simulink library "lidar_script_other_ver"  (R2021a)
settings: Solver=VariableStepAuto  StartTime=0.0  StopTime=10.0  RelTol=1e-3
undefined symbols (not defined in the file or in its folder): sim3d
settings Model: ModifiedByFormat=The MathWorks, Inc.  Creator=The MathWorks, Inc.  LastModifiedBy=The MathWorks, Inc.
settings SolverCC: AlgebraicLoopSolver=TrustRegion
settings DebuggingCC: SFMachineParentedDataDiag=warning

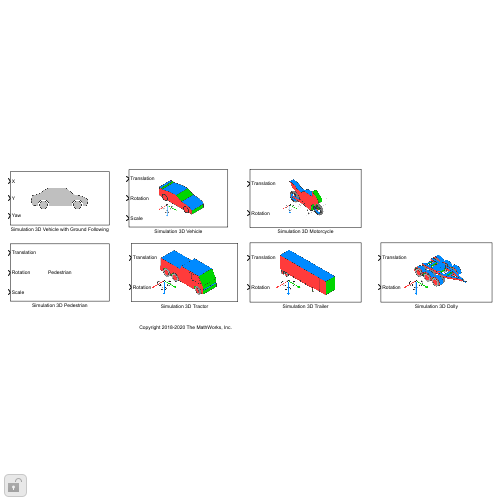
[thumbnail: Simulink's stored preview of the top-level diagram]
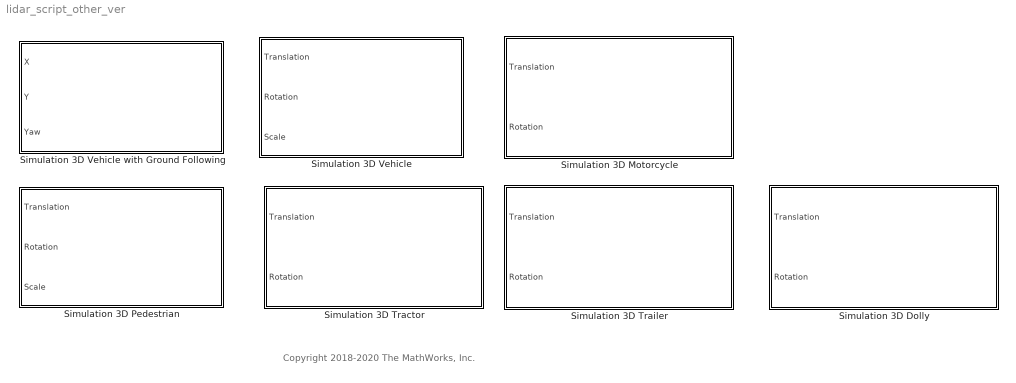
== system lidar_script_other_ver ==
  note: Copyright 2018-2020 The MathWorks, Inc.
  Simulation 3D Dolly : Subsystem  Priority=-1  LoadFcn=sim3d.SimPool.loadCallback(gcb)  mask(Simulation 3D Dolly){Mesh=One-axle dolly, Mesh_Internal=One-axle dolly, ActorName=, Translation=zeros( 5, 3 ), Rotation=zeros( 5, 3 ), Scale=ones( 5, 3 ), SampleTime=-1, ActorType=SimulinkVehicle, ID=[], aMode=aMode, ActorTag=}
      mask prompts: Mesh "shared_sim3dblks:sim3dblkDolly:blkPrm_Mesh"; Mesh_Internal "shared_sim3dblks:sim3dblkDolly:blkPrm_Mesh"; ActorName "shared_sim3dblks:sim3dblkDolly:blkPrm_ActorName"; Translation "shared_sim3dblks:sim3dblkDolly:blkPrm_Translation"; Rotation "shared_sim3dblks:sim3dblkDolly:blkPrm_Rotation"; SampleTime "shared_sim3dblks:sim3dblkDolly:blkPrm_SampleTime"
      mask help: shared_sim3dblks:sim3dblkDolly:blkDesc
      mask init:
      | sim3dblkssharedicon('sim3dblksdolly',gcb,'Initialization');
      settings: CopyFcn=sim3d.SimPool.copyCallback(gcb);  UndoDeleteFcn=sim3d.SimPool.UndoDeleteCallback(gcb)  PostSaveFcn=sim3d.SimPool.postSaveCallback(gcb)  NameChangeFcn=sim3d.SimPool.nameChangeCallback(gcb)  DestroyFcn=sim3d.SimPool.DestroyCallback(gcb)  PreDeleteFcn=sim3d.SimPool.preDeleteCallback(gcb);
      mask Help: eval('sim3dblkssharedhelp(''sim3ddolly'')');
      mask TypeOptions Mesh: shared_sim3dblks:sim3dblkDolly:oneaxledolly | shared_sim3dblks:sim3dblkDolly:twoaxledolly | shared_sim3dblks:sim3dblkDolly:threeaxledolly
      mask TypeOptions Mesh_Internal: Simulation 3D Dolly/Mesh
      mask Callback Mesh_Internal: sim3dblkssharedicon('sim3dblksdolly',gcb,'SetInitialValues');
      mask TypeOptions Translation: Simulation 3D Dolly/Translation
      mask TypeOptions Rotation: Simulation 3D Dolly/Rotation
      mask TypeOptions Scale: Simulation 3D Dolly/Scale
      mask TypeOptions SampleTime: Simulation 3D Dolly/SampleTime
      mask DialogControl ParameterGroupVar Prompt: shared_sim3dblks:sim3dblkDolly:blkDlg_ParameterGroupVar
      mask DialogControl Mesh Prompt: Type:
      mask DialogControl Mesh_Internal Prompt: Type:
      mask DialogControl ActorName Prompt: Name:
      mask DialogControl Container5 Prompt: shared_sim3dblks:sim3dblkDolly:blkDlg_Container5
      mask DialogControl Translation Prompt: Initial array values to translate vehicle per part, Translation (m):
      mask DialogControl Rotation Prompt: Initial array values to rotate vehicle per part, Rotation (rad):
      mask DialogControl SampleTime Prompt: Sample time:
      mask Display:
      | IconInfo = sim3dblkssharedicon('sim3dblksdolly', gcb, 'DrawCommands');
      | 
      | image(IconInfo.image, IconInfo.position);
      | 
      | for i = 1:numel(IconInfo.lconn)
      |     port_label('lconn', i, IconInfo.lconn{i})
      | end
      | 
      | for j = 1:numel(IconInfo.rconn)
      |     port_label('rconn', j, IconInfo.rconn{j})
      | end
      | 
      | for k = 1:numel(IconInfo.input)
      |     port_label('input', k, IconInfo.input{k})
      | end
      | 
      | for m = 1:numel(IconInfo.output)
      |     port_label('output', m, IconInfo.output{m})
      | end
  Simulation 3D Motorcycle : Subsystem  Priority=-1  LoadFcn=sim3d.SimPool.loadCallback(gcb)  mask(Simulation 3D Motorcycle){Mesh=Sports bike, Mesh_Internal=Sports bike, MotorcycleColor=Red, MotorcycleColor_Internal=Red, ActorName=, Translation=zeros( 4, 3 ), Rotation=zeros( 4, 3 ), SampleTime=-1, ActorType=SimulinkVehicle, ID=[], aMode=aMode, ActorTag=}
      mask prompts: Mesh "shared_sim3dblks:sim3dblkMotorcycle:blkPrm_Mesh"; Mesh_Internal "shared_sim3dblks:sim3dblkMotorcycle:blkPrm_Mesh"; MotorcycleColor "shared_sim3dblks:sim3dblkMotorcycle:blkPrm_Color"; MotorcycleColor_Internal "shared_sim3dblks:sim3dblkMotorcycle:blkPrm_Color"; ActorName "shared_sim3dblks:sim3dblkMotorcycle:blkPrm_ActorName"; Translation "shared_sim3dblks:sim3dblkMotorcycle:blkPrm_Translation"; Rotation "shared_sim3dblks:sim3dblkMotorcycle:blkPrm_Rotation"; SampleTime "shared_sim3dblks:sim3dblkMotorcycle:blkPrm_SampleTime"
      mask help: shared_sim3dblks:sim3dblkMotorcycle:blkDesc
      mask init:
      | sim3dblkssharedicon('sim3dblksmotorcycle',gcb,'Initialization');
      settings: CopyFcn=sim3d.SimPool.copyCallback(gcb);  UndoDeleteFcn=sim3d.SimPool.UndoDeleteCallback(gcb)  PostSaveFcn=sim3d.SimPool.postSaveCallback(gcb)  NameChangeFcn=sim3d.SimPool.nameChangeCallback(gcb)  DestroyFcn=sim3d.SimPool.DestroyCallback(gcb)  PreDeleteFcn=sim3d.SimPool.preDeleteCallback(gcb);
      mask Help: eval('sim3dblkssharedhelp(''sim3dmotorcycle'')');
      mask TypeOptions Mesh: shared_sim3dblks:sim3dblkMotorcycle:sports | shared_sim3dblks:sim3dblkMotorcycle:economy | shared_sim3dblks:sim3dblkMotorcycle:scooter
      mask TypeOptions Mesh_Internal: Simulation 3D Motorcycle/Mesh
      mask TypeOptions MotorcycleColor: shared_sim3dblks:sim3dblkMotorcycle:red | shared_sim3dblks:sim3dblkMotorcycle:orange | shared_sim3dblks:sim3dblkMotorcycle:yellow | shared_sim3dblks:sim3dblkMotorcycle:blue | shared_sim3dblks:sim3dblkMotorcycle:green | shared_sim3dblks:sim3dblkMotorcycle:white | shared_sim3dblks:sim3dblkMotorcycle:black | shared_sim3dblks:sim3dblkMotorcycle:silver
      mask TypeOptions MotorcycleColor_Internal: Simulation 3D Motorcycle/MotorcycleColor
      mask TypeOptions Translation: Simulation 3D Motorcycle/Translation
      mask TypeOptions Rotation: Simulation 3D Motorcycle/Rotation
      mask TypeOptions SampleTime: Simulation 3D Motorcycle/SampleTime
      mask DialogControl Container4 Prompt: Vehicle Parameters
      mask DialogControl Mesh Prompt: Type:
      mask DialogControl Mesh_Internal Prompt: Type:
      mask DialogControl MotorcycleColor Prompt: Color:
      mask DialogControl MotorcycleColor_Internal Prompt: Color:
      mask DialogControl ActorName Prompt: Name:
      mask DialogControl Container5 Prompt: shared_sim3dblks:sim3dblkMotorcycle:blkDlg_Container5
      mask DialogControl Translation Prompt: Initial array values to translate vehicle per part, Translation (m):
      mask DialogControl Rotation Prompt: Initial array values to rotate vehicle per part, Rotation (rad):
      mask DialogControl SampleTime Prompt: Sample time:
      mask Display:
      | IconInfo = sim3dblkssharedicon('sim3dblksmotorcycle', gcb, 'DrawCommands');
      | 
      | image(IconInfo.image, IconInfo.position);
      | 
      | for i = 1:numel(IconInfo.lconn)
      |     port_label('lconn', i, IconInfo.lconn{i})
      | end
      | 
      | for j = 1:numel(IconInfo.rconn)
      |     port_label('rconn', j, IconInfo.rconn{j})
      | end
      | 
      | for k = 1:numel(IconInfo.input)
      |     port_label('input', k, IconInfo.input{k})
      | end
      | 
      | for m = 1:numel(IconInfo.output)
      |     port_label('output', m, IconInfo.output{m})
      | end
  Simulation 3D Pedestrian : Subsystem  Priority=-1  LoadFcn=sim3d.SimPool.loadCallback(gcb)  mask(Simulation 3D Pedestrian){PassVehMesh=Hatchback, VehColor=Red, ZoffsetPos=0, ActorName=, SampleTime=-1, ActorType=Pedestrian, ID=1, aMode=aMode, ActorTag=Pedestrian1}
      mask prompts: PassVehMesh "Type:"; VehColor "Color:"; ZoffsetPos "Initial Z position:"; ActorName "Name:"; SampleTime "Sample time:"
      mask help: Implements a pedestrian in the 3D visualization environment. The block uses the pedestrian translation, rotation, and scale to position the pedestrian in the 3D environment. Depending on the rate of change of the position, the block implements a pedestrian that walks or runs.
      mask init:
      | P = sim3dblkssharedicon('sim3dblks3dped',gcb,'Initialization');
      settings: CopyFcn=sim3d.SimPool.copyCallback(gcb);  UndoDeleteFcn=sim3d.SimPool.UndoDeleteCallback(gcb)  PostSaveFcn=sim3d.SimPool.postSaveCallback(gcb)  NameChangeFcn=sim3d.SimPool.nameChangeCallback(gcb)  DestroyFcn=sim3d.SimPool.DestroyCallback(gcb)  PreDeleteFcn=sim3d.SimPool.preDeleteCallback(gcb);
      mask Help: eval('sim3dblkssharedhelp(''sim3dpedestrian'')');
      mask TypeOptions PassVehMesh: Simulation 3D Pedestrian/PassVehMesh
      mask TypeOptions VehColor: Simulation 3D Pedestrian/VehColor
      mask TypeOptions ZoffsetPos: Simulation 3D Pedestrian/ZoffsetPos
      mask TypeOptions SampleTime: Simulation 3D Pedestrian/SampleTime | PlantParser/Passenger Vehicle Ray Trace Set/Ts
      mask DialogControl ParameterGroupVar Prompt: Vehicle Parameters
      mask Display:
      | IconInfo = sim3dblkssharedicon('sim3dblks3dped', gcb, 'DrawCommands');
      | 
      | %% The next two lines are mutually exclusive
      | % image(IconInfo.image, IconInfo.position);
      | disp('Pedestrian')
      | 
      | for i = 1:numel(IconInfo.lconn)
      |     port_label('lconn', i, IconInfo.lconn{i})
      | end
      | 
      | for j = 1:numel(IconInfo.rconn)
      |     port_label('rconn', j, IconInfo.rconn{j})
      | end
      | 
      | for k = 1:numel(IconInfo.input)
      |     port_label('input', k, IconInfo.input{k})
      | end
      | 
      | for m = 1:numel(IconInfo.output)
      |     port_label('output', m, IconInfo.output{m})
      | end
  Simulation 3D Tractor : Subsystem  Priority=-1  LoadFcn=sim3d.SimPool.loadCallback(gcb)  mask(Simulation 3D Tractor){Mesh=Conventional tractor, Mesh_Internal=Conventional tractor, TractorColor=Red, TractorColor_Internal=Red, ActorName=, Translation=zeros( 7, 3 ), Rotation=zeros( 7, 3 ), SampleTime=-1, ActorType=SimulinkVehicle, ID=[], aMode=aMode, ActorTag=}
      mask prompts: Mesh "shared_sim3dblks:sim3dblkTractor:blkPrm_Mesh"; Mesh_Internal "shared_sim3dblks:sim3dblkTractor:blkPrm_Mesh"; TractorColor "shared_sim3dblks:sim3dblkTractor:blkPrm_Color"; TractorColor_Internal "shared_sim3dblks:sim3dblkTractor:blkPrm_Color"; ActorName "shared_sim3dblks:sim3dblkTractor:blkPrm_ActorName"; Translation "shared_sim3dblks:sim3dblkTractor:blkPrm_Translation"; Rotation "shared_sim3dblks:sim3dblkTractor:blkPrm_Rotation"; SampleTime "shared_sim3dblks:sim3dblkTractor:blkPrm_SampleTime"
      mask help: shared_sim3dblks:sim3dblkTractor:blkDesc
      mask init:
      | sim3dblkssharedicon('sim3dblkstractor',gcb,'Initialization');
      settings: CopyFcn=sim3d.SimPool.copyCallback(gcb);  UndoDeleteFcn=sim3d.SimPool.UndoDeleteCallback(gcb)  PostSaveFcn=sim3d.SimPool.postSaveCallback(gcb)  NameChangeFcn=sim3d.SimPool.nameChangeCallback(gcb)  DestroyFcn=sim3d.SimPool.DestroyCallback(gcb)  PreDeleteFcn=sim3d.SimPool.preDeleteCallback(gcb);
      mask Help: eval('sim3dblkssharedhelp(''sim3dtractor'')');
      mask TypeOptions Mesh: shared_sim3dblks:sim3dblkTractor:conventionaltractor | shared_sim3dblks:sim3dblkTractor:cabovertractor
      mask TypeOptions Mesh_Internal: Simulation 3D Tractor/Mesh
      mask TypeOptions TractorColor: shared_sim3dblks:sim3dblkTractor:red | shared_sim3dblks:sim3dblkTractor:orange | shared_sim3dblks:sim3dblkTractor:yellow | shared_sim3dblks:sim3dblkTractor:blue | shared_sim3dblks:sim3dblkTractor:green | shared_sim3dblks:sim3dblkTractor:white | shared_sim3dblks:sim3dblkTractor:black | shared_sim3dblks:sim3dblkTractor:silver
      mask TypeOptions TractorColor_Internal: Simulation 3D Tractor/TractorColor
      mask TypeOptions Translation: Simulation 3D Tractor/Translation
      mask TypeOptions Rotation: Simulation 3D Tractor/Rotation
      mask TypeOptions SampleTime: Simulation 3D Tractor/SampleTime
      mask DialogControl ParameterGroupVar Prompt: shared_sim3dblks:sim3dblkTractor:blkDlg_ParameterGroupVar
      mask DialogControl Mesh Prompt: Type:
      mask DialogControl Mesh_Internal Prompt: Type:
      mask DialogControl TractorColor Prompt: Color:
      mask DialogControl TractorColor_Internal Prompt: Color:
      mask DialogControl ActorName Prompt: Name:
      mask DialogControl Container4 Prompt: shared_sim3dblks:sim3dblkTractor:blkDlg_Container5
      mask DialogControl Translation Prompt: Initial array values to translate vehicle per part, Translation (m):
      mask DialogControl Rotation Prompt: Initial array values to rotate vehicle per part, Rotation (rad):
      mask DialogControl SampleTime Prompt: Sample time:
      mask Display:
      | IconInfo = sim3dblkssharedicon('sim3dblkstractor', gcb, 'DrawCommands');
      | 
      | image(IconInfo.image, IconInfo.position);
      | 
      | for i = 1:numel(IconInfo.lconn)
      |     port_label('lconn', i, IconInfo.lconn{i})
      | end
      | 
      | for j = 1:numel(IconInfo.rconn)
      |     port_label('rconn', j, IconInfo.rconn{j})
      | end
      | 
      | for k = 1:numel(IconInfo.input)
      |     port_label('input', k, IconInfo.input{k})
      | end
      | 
      | for m = 1:numel(IconInfo.output)
      |     port_label('output', m, IconInfo.output{m})
      | end
  Simulation 3D Trailer : Subsystem  Priority=-1  LoadFcn=sim3d.SimPool.loadCallback(gcb)  mask(Simulation 3D Trailer){Mesh=Two-axle trailer, Mesh_Internal=Two-axle trailer, ActorName=, Translation=zeros(5,3), Rotation=zeros(5,3), SampleTime=-1, ActorType=SimulinkVehicle, ID=[], aMode=aMode, ActorTag=}
      mask prompts: Mesh "shared_sim3dblks:sim3dblkTrailer:blkPrm_Mesh"; Mesh_Internal "shared_sim3dblks:sim3dblkTrailer:blkPrm_Mesh"; ActorName "shared_sim3dblks:sim3dblkTrailer:blkPrm_ActorName"; Translation "shared_sim3dblks:sim3dblkTrailer:blkPrm_Translation"; Rotation "shared_sim3dblks:sim3dblkTrailer:blkPrm_Rotation"; SampleTime "shared_sim3dblks:sim3dblkTrailer:blkPrm_SampleTime"
      mask help: shared_sim3dblks:sim3dblkTrailer:blkDesc
      mask init:
      | sim3dblkssharedicon('sim3dblkstrailer',gcb,'Initialization');
      settings: CopyFcn=sim3d.SimPool.copyCallback(gcb);  UndoDeleteFcn=sim3d.SimPool.UndoDeleteCallback(gcb)  PostSaveFcn=sim3d.SimPool.postSaveCallback(gcb)  NameChangeFcn=sim3d.SimPool.nameChangeCallback(gcb)  DestroyFcn=sim3d.SimPool.DestroyCallback(gcb)  PreDeleteFcn=sim3d.SimPool.preDeleteCallback(gcb);
      mask Help: eval('sim3dblkssharedhelp(''sim3dtrailer'')');
      mask TypeOptions Mesh: shared_sim3dblks:sim3dblkTrailer:twoaxletrailer | shared_sim3dblks:sim3dblkTrailer:threeaxletrailer
      mask TypeOptions Mesh_Internal: Simulation 3D Trailer/Mesh
      mask Callback Mesh_Internal: sim3dblkssharedicon('sim3dblkstrailer',gcb,'SetInitialValues');
      mask TypeOptions Translation: Simulation 3D Dolly/Translation
      mask TypeOptions Rotation: Simulation 3D Dolly/Rotation
      mask TypeOptions SampleTime: Simulation 3D Dolly/SampleTime
      mask DialogControl ParameterGroupVar Prompt: shared_sim3dblks:sim3dblkTrailer:blkDlg_ParameterGroupVar
      mask DialogControl Mesh Prompt: Type:
      mask DialogControl Mesh_Internal Prompt: Type:
      mask DialogControl ActorName Prompt: Name:
      mask DialogControl Container5 Prompt: shared_sim3dblks:sim3dblkTrailer:blkDlg_Container5
      mask DialogControl Translation Prompt: Initial array values to translate vehicle per part, Translation (m):
      mask DialogControl Rotation Prompt: Initial array values to rotate vehicle per part, Rotation (rad):
      mask DialogControl SampleTime Prompt: Sample time:
      mask Display:
      | IconInfo = sim3dblkssharedicon('sim3dblkstrailer', gcb, 'DrawCommands');
      | 
      | image(IconInfo.image, IconInfo.position);
      | 
      | for i = 1:numel(IconInfo.lconn)
      |     port_label('lconn', i, IconInfo.lconn{i})
      | end
      | 
      | for j = 1:numel(IconInfo.rconn)
      |     port_label('rconn', j, IconInfo.rconn{j})
      | end
      | 
      | for k = 1:numel(IconInfo.input)
      |     port_label('input', k, IconInfo.input{k})
      | end
      | 
      | for m = 1:numel(IconInfo.output)
      |     port_label('output', m, IconInfo.output{m})
      | end
  Simulation 3D Vehicle : Subsystem  Priority=-1  LoadFcn=sim3d.SimPool.loadCallback(gcb)  mask(Simulation 3D Vehicle){PassVehMesh=Muscle car, PassVehMesh_Internal=Muscle car, MeshPath=/MathWorksSimulation/Vehicles/Muscle/Meshes/SK_MuscleCar.SK_MuscleCar, VehColor=Red, VehColor_Internal=Red, ActorName=, VehLightsControl=off, HeadlightColor=[ 1, 1, 1 ], HighBeamIntensity=100000, LowBeamIntensity=60000, HighBeamConeAngle=1.22, LowBeamConeAngle=1.22, LeftHeadlightOrientation=[ 0, 0 ], RightHeadlightOrientation=[ 0, 0 ], BrakelightIntensity=500, ReverselightIntensity=500, SignallightIntensity=500, SignallightPeriod=1, SignalPulseWidth=50, Translation=zeros( 5, 3 ), Rotation=zeros( 5, 3 ), Scale=ones( 5, 3 ), SampleTime=-1, ActorType=SimulinkVehicle, ID=, aMode=aMode, ActorTag=}
      mask prompts: PassVehMesh "shared_sim3dblks:sim3dblkVehicle:blkPrm_PassVehMesh"; PassVehMesh_Internal "shared_sim3dblks:sim3dblkVehicle:blkPrm_PassVehMesh"; MeshPath "shared_sim3dblks:sim3dblkVehicle:blkPrm_MeshPath"; VehColor "shared_sim3dblks:sim3dblkVehicle:blkPrm_VehColor"; VehColor_Internal "shared_sim3dblks:sim3dblkVehicle:blkPrm_VehColor"; ActorName "shared_sim3dblks:sim3dblkVehicle:blkPrm_ActorName"; VehLightsControl "shared_sim3dblks:sim3dblkVehicle:blkPrm_VehLightsControl"; HeadlightColor "shared_sim3dblks:sim3dblkVehicle:blkPrm_HeadlightColor"; HighBeamIntensity "shared_sim3dblks:sim3dblkVehicle:blkPrm_HighBeamIntensity"; LowBeamIntensity "shared_sim3dblks:sim3dblkVehicle:blkPrm_LowBeamIntensity"; HighBeamConeAngle "shared_sim3dblks:sim3dblkVehicle:blkPrm_HighBeamRadius"; LowBeamConeAngle "shared_sim3dblks:sim3dblkVehicle:blkPrm_LowBeamRadius"; LeftHeadlightOrientation "shared_sim3dblks:sim3dblkVehicle:blkPrm_LeftBeamOrientation"; RightHeadlightOrientation "shared_sim3dblks:sim3dblkVehicle:blkPrm_RightBeamOrientation"; BrakelightIntensity "shared_sim3dblks:sim3dblkVehicle:blkPrm_BrakelightIntensity"; ReverselightIntensity "shared_sim3dblks:sim3dblkVehicle:blkPrm_ReverselightIntensity"; SignallightIntensity "shared_sim3dblks:sim3dblkVehicle:blkPrm_SignallightIntensity"; SignallightPeriod "shared_sim3dblks:sim3dblkVehicle:blkPrm_SignalPeriod"; SignalPulseWidth "shared_sim3dblks:sim3dblkVehicle:blkPrm_SignalPulseWidth"; Translation "shared_sim3dblks:sim3dblkVehicle:blkPrm_Translation"; Rotation "shared_sim3dblks:sim3dblkVehicle:blkPrm_Rotation"; Scale "shared_sim3dblks:sim3dblkVehicle:blkPrm_Scale"; SampleTime "shared_sim3dblks:sim3dblkVehicle:blkPrm_SampleTime"
      mask help: shared_sim3dblks:sim3dblkVehicle:blkDesc
      mask init:
      | sim3dblkssharedicon('sim3dblks3dveh',gcb,'Initialization');
      settings: CopyFcn=sim3d.SimPool.copyCallback(gcb);  UndoDeleteFcn=sim3d.SimPool.UndoDeleteCallback(gcb)  PostSaveFcn=sim3d.SimPool.postSaveCallback(gcb)  NameChangeFcn=sim3d.SimPool.nameChangeCallback(gcb)  DestroyFcn=sim3d.SimPool.DestroyCallback(gcb)  PreDeleteFcn=sim3d.SimPool.preDeleteCallback(gcb);
      mask Help: eval('sim3dblkssharedhelp(''sim3dvehicle'')');
      mask TypeOptions PassVehMesh: shared_sim3dblks:sim3dblkVehicle:musclecar | shared_sim3dblks:sim3dblkVehicle:sedan | shared_sim3dblks:sim3dblkVehicle:sportutilityvehicle | shared_sim3dblks:sim3dblkVehicle:smallpickuptruck | shared_sim3dblks:sim3dblkVehicle:hatchback | shared_sim3dblks:sim3dblkVehicle:boxtruck | shared_sim3dblks:sim3dblkVehicle:custom
      mask Callback PassVehMesh: sim3dblkssharedicon('sim3dblks3dveh',gcb,'VehicleSelection');
      mask TypeOptions PassVehMesh_Internal: Simulation 3D Vehicle/PassVehMesh
      mask TypeOptions VehColor: shared_sim3dblks:sim3dblkVehicle:red | shared_sim3dblks:sim3dblkVehicle:orange | shared_sim3dblks:sim3dblkVehicle:yellow | shared_sim3dblks:sim3dblkVehicle:blue | shared_sim3dblks:sim3dblkVehicle:green | shared_sim3dblks:sim3dblkVehicle:white | shared_sim3dblks:sim3dblkVehicle:black | shared_sim3dblks:sim3dblkVehicle:silver
      mask TypeOptions VehColor_Internal: Simulation 3D Vehicle/VehColor
      mask Callback VehLightsControl: sim3dblkssharedicon('sim3dblks3dveh',gcb,'VehLightsControl');
      mask TypeOptions HeadlightColor: Simulation 3D Vehicle/HeadligtColor
      mask TypeOptions HighBeamIntensity: Simulation 3D Vehicle/HighBeamIntensity
      mask TypeOptions LowBeamIntensity: Simulation 3D Vehicle/LowBeamIntensity
      mask TypeOptions HighBeamConeAngle: Simulation 3D Vehicle/HighBeamRadius
      mask TypeOptions LowBeamConeAngle: Simulation 3D Vehicle/LowBeamRadius
      mask TypeOptions LeftHeadlightOrientation: Simulation 3D Vehicle/LeftHeadlightOrientation
      mask TypeOptions RightHeadlightOrientation: Simulation 3D Vehicle/RightHeadlightOrientation
      mask TypeOptions BrakelightIntensity: Simulation 3D Vehicle/BrakelightIntensity
      mask TypeOptions ReverselightIntensity: Simulation 3D Vehicle/ReverselightIntensity
      mask TypeOptions SignallightIntensity: Simulation 3D Vehicle/IndicatorlightIntensity
      mask TypeOptions SignallightPeriod:
      | Signal Lights Processor/Pulse
      | Generator/Period
      mask TypeOptions SignalPulseWidth:
      | Signal Lights Processor/Pulse
      | Generator/PulseWidth
      mask TypeOptions Translation: Simulation 3D Vehicle/Translation
      mask TypeOptions Rotation: Simulation 3D Vehicle/Rotation
      mask TypeOptions Scale: Simulation 3D Vehicle/Scale
      mask TypeOptions SampleTime: Simulation 3D Vehicle/SampleTime
      mask DialogControl ParameterGroupVar Prompt: shared_sim3dblks:sim3dblkVehicle:blkDlg_ParameterGroupVar
      mask DialogControl PassVehMesh Prompt: Type, PassVehMesh:
      mask DialogControl PassVehMesh_Internal Prompt: Type, PassVehMesh:
      mask DialogControl MeshPath Prompt: Path to custom mesh, MeshPath:
      mask DialogControl VehColor Prompt: Color, VehColor:
      mask DialogControl VehColor_Internal Prompt: Color, VehColor:
      mask DialogControl ActorName Prompt: Name, ActorName:
      mask DialogControl VehLightsTab Prompt: shared_sim3dblks:sim3dblkVehicle:blkDg_LightControlsTab
      mask DialogControl VehLightsControl Prompt: Enable light controls, VehLightsControl:
      mask DialogControl HeadlightSettingsMenu Prompt: shared_sim3dblks:sim3dblkVehicle:blkPrm_HeadlightSettings
      mask DialogControl HeadlightColor Prompt: Headlight color [R,G,B], HeadlightColor:
      mask DialogControl HighBeamIntensity Prompt: High beam intensity, HighBeamIntensity [cd]:
      mask DialogControl LowBeamIntensity Prompt: Low beam intensity, LowBeamIntensity [cd]:
      mask DialogControl HighBeamConeAngle Prompt: High beam cone half angle, HighBeamConeAngle [rad]:
      mask DialogControl LowBeamConeAngle Prompt: Low beam cone half angle, LowBeamConeAngle [rad]:
      mask DialogControl LeftHeadlightOrientation Prompt: Left headlight beam orientation [Pitch, Yaw], LeftHeadlightOrientation [rad]:
      mask DialogControl RightHeadlightOrientation Prompt: Right headlight beam orientation [Pitch, Yaw], RightHeadlightOrientation [rad]:
      mask DialogControl BrakelightSettingsMenu Prompt: shared_sim3dblks:sim3dblkVehicle:blkPrm_BrakelightSettings
      mask DialogControl BrakelightIntensity Prompt: Brake light intensity, BrakelightIntensity [cd/m^2]:
      mask DialogControl ReverselightSettingsMenu Prompt: shared_sim3dblks:sim3dblkVehicle:blkPrm_ReverselightSettings
      mask DialogControl ReverselightIntensity Prompt: Reverse light intensity, ReverselightIntensity [cd/m^2]:
      mask DialogControl SignallightSettingsMenu Prompt: shared_sim3dblks:sim3dblkVehicle:blkPrm_SignallightSettings
      mask DialogControl SignallightIntensity Prompt: Turn signal light intensity, SignallightIntensity [cd/m^2]:
      mask DialogControl SignallightPeriod Prompt: Period, SignallightPeriod [s]:
      mask DialogControl SignalPulseWidth Prompt: Pulse width, SignalPulseWidth [% of period]:
      mask DialogControl Container5 Prompt: shared_sim3dblks:sim3dblkVehicle:blkDlg_Container5
      mask DialogControl Translation Prompt: Initial array values to translate vehicle per part, Translation (m):
      mask DialogControl Rotation Prompt: Initial array values to rotate vehicle per part, Rotation (rad):
      mask DialogControl Scale Prompt: Initial array values to scale vehicle per part, Scale:
      mask DialogControl SampleTime Prompt: Sample time, SampleTime:
      mask Display:
      | IconInfo = sim3dblkssharedicon('sim3dblks3dveh', gcb, 'DrawCommands');
      | 
      | image(IconInfo.image, IconInfo.position);
      | 
      | for i = 1:numel(IconInfo.lconn)
      |     port_label('lconn', i, IconInfo.lconn{i})
      | end
      | 
      | for j = 1:numel(IconInfo.rconn)
      |     port_label('rconn', j, IconInfo.rconn{j})
      | end
      | 
      | for k = 1:numel(IconInfo.input)
      |     port_label('input', k, IconInfo.input{k})
      | end
      | 
      | for m = 1:numel(IconInfo.output)
      |     port_label('output', m, IconInfo.output{m})
      | end
  Simulation 3D Vehicle with Ground Following : Subsystem  Priority=-1  LoadFcn=sim3d.SimPool.loadCallback(gcb)  mask(Simulation 3D Vehicle with Ground Following){PassVehMesh=Muscle car, PassVehMesh_Internal=Muscle car, MeshPath=/MathWorksSimulation/Vehicles/Muscle/Meshes/SK_MuscleCar.SK_MuscleCar, TrackWidth=1.9, WheelBase=3, WheelRadius=0.35, VehColor=Red, VehColor_Internal=Red, InitialPos=[0, 0, 0], InitialRot=[0, 0, 0], ActorName=, SampleTime=-1, ActorType=SimulinkVehicle, ID=1, aMode=aMode, ActorTag=SimulinkVehicle1, CoordinateScheme=ISO, VehLightsControl=off, HeadlightColor=[ 1, 1, 1 ], HighBeamIntensity=100000, LowBeamIntensity=60000, HighBeamConeAngle=70, LowBeamConeAngle=70, LeftHeadlightOrientation=[ 0, 0 ], RightHeadlightOrientation=[ 0, 0 ], BrakelightIntensity=500, ReverselightIntensity=500, SignallightIntensity=500, SignallightPeriod=1, SignalPulseWidth=50, TransformOutportEnabled=off}
      mask prompts: PassVehMesh "shared_sim3dblks:sim3dblkVehicleWithGroundFollowing:blkPrm_PassVehMesh"; PassVehMesh_Internal "shared_sim3dblks:sim3dblkVehicleWithGroundFollowing:blkPrm_PassVehMesh"; MeshPath "shared_sim3dblks:sim3dblkVehicleWithGroundFollowing:blkPrm_MeshPath"; TrackWidth "shared_sim3dblks:sim3dblkVehicleWithGroundFollowing:blkPrm_TrackWidth"; WheelBase "shared_sim3dblks:sim3dblkVehicleWithGroundFollowing:blkPrm_WheelBase"; WheelRadius "shared_sim3dblks:sim3dblkVehicleWithGroundFollowing:blkPrm_WheelRadius"; VehColor "shared_sim3dblks:sim3dblkVehicleWithGroundFollowing:blkPrm_VehColor"; VehColor_Internal "shared_sim3dblks:sim3dblkVehicleWithGroundFollowing:blkPrm_VehColor"; InitialPos "shared_sim3dblks:sim3dblkVehicleWithGroundFollowing:blkPrm_InitialPos"; InitialRot "shared_sim3dblks:sim3dblkVehicleWithGroundFollowing:blkPrm_InitialRotISO"; ActorName "shared_sim3dblks:sim3dblkVehicleWithGroundFollowing:blkPrm_ActorName"; SampleTime "shared_sim3dblks:sim3dblkVehicleWithGroundFollowing:blkPrm_SampleTime"; CoordinateScheme "shared_sim3dblks:sim3dblkVehicleWithGroundFollowing:blkPrm_CoordinateScheme"; VehLightsControl "shared_sim3dblks:sim3dblkVehicleWithGroundFollowing:blkPrm_VehLightsControl"; HeadlightColor "shared_sim3dblks:sim3dblkVehicleWithGroundFollowing:blkPrm_HeadlightColor"; HighBeamIntensity "shared_sim3dblks:sim3dblkVehicleWithGroundFollowing:blkPrm_HighBeamIntensity"; LowBeamIntensity "shared_sim3dblks:sim3dblkVehicleWithGroundFollowing:blkPrm_LowBeamIntensity"; HighBeamConeAngle "shared_sim3dblks:sim3dblkVehicleWithGroundFollowing:blkPrm_HighBeamRadius"; LowBeamConeAngle "shared_sim3dblks:sim3dblkVehicleWithGroundFollowing:blkPrm_LowBeamRadius"; LeftHeadlightOrientation "shared_sim3dblks:sim3dblkVehicleWithGroundFollowing:blkPrm_LeftBeamOrientation"; RightHeadlightOrientation "shared_sim3dblks:sim3dblkVehicleWithGroundFollowing:blkPrm_RightBeamOrientation"; BrakelightIntensity "shared_sim3dblks:sim3dblkVehicleWithGroundFollowing:blkPrm_BrakelightIntensity"; ReverselightIntensity "shared_sim3dblks:sim3dblkVehicleWithGroundFollowing:blkPrm_ReverselightIntensity"; SignallightIntensity "shared_sim3dblks:sim3dblkVehicleWithGroundFollowing:blkPrm_SignallightIntensity"; SignallightPeriod "shared_sim3dblks:sim3dblkVehicleWithGroundFollowing:blkPrm_SignalPeriod"; SignalPulseWidth "shared_sim3dblks:sim3dblkVehicleWithGroundFollowing:blkPrm_SignalPulseWidth"; TransformOutportEnabled "shared_sim3dblks:sim3dblkVehicleWithGroundFollowing:blkPrm_TransformOutputEnabled"
      mask help: shared_sim3dblks:sim3dblkVehicleWithGroundFollowing:blkDesc
      mask init:
      | P = sim3dblkssharedicon('sim3dblks3dvehterrfb',gcb,'Initialization');
      settings: CopyFcn=sim3d.SimPool.copyCallback(gcb);  UndoDeleteFcn=sim3d.SimPool.UndoDeleteCallback(gcb)  PostSaveFcn=sim3d.SimPool.postSaveCallback(gcb)  NameChangeFcn=sim3d.SimPool.nameChangeCallback(gcb)  DestroyFcn=sim3d.SimPool.DestroyCallback(gcb)  PreDeleteFcn=sim3d.SimPool.preDeleteCallback(gcb);
      mask Help: eval('sim3dblkssharedhelp(''sim3dvehiclefollowing'')');
      mask TypeOptions PassVehMesh: shared_sim3dblks:sim3dblkVehicleWithGroundFollowing:musclecar | shared_sim3dblks:sim3dblkVehicleWithGroundFollowing:sedan | shared_sim3dblks:sim3dblkVehicleWithGroundFollowing:sportutilityvehicle | shared_sim3dblks:sim3dblkVehicleWithGroundFollowing:smallpickuptruck | shared_sim3dblks:sim3dblkVehicleWithGroundFollowing:hatchback | shared_sim3dblks:sim3dblkVehicleWithGroundFollowing:boxtruck | shared_sim3dblks:sim3dblkVehicleWithGroundFollowing:custom
      mask Callback PassVehMesh: sim3dblkssharedicon('sim3dblks3dvehterrfb',gcb,'VehicleSelection');
      mask TypeOptions PassVehMesh_Internal: Simulation 3D Vehicle/PassVehMesh
      mask TypeOptions VehColor: shared_sim3dblks:sim3dblkVehicleWithGroundFollowing:red | shared_sim3dblks:sim3dblkVehicleWithGroundFollowing:orange | shared_sim3dblks:sim3dblkVehicleWithGroundFollowing:yellow | shared_sim3dblks:sim3dblkVehicleWithGroundFollowing:blue | shared_sim3dblks:sim3dblkVehicleWithGroundFollowing:green | shared_sim3dblks:sim3dblkVehicleWithGroundFollowing:white | shared_sim3dblks:sim3dblkVehicleWithGroundFollowing:black | shared_sim3dblks:sim3dblkVehicleWithGroundFollowing:silver
      mask TypeOptions VehColor_Internal: Simulation 3D Vehicle/VehColor
      mask TypeOptions InitialPos: Simulation 3D Vehicle/InitialPos
      mask TypeOptions InitialRot: Simulation 3D Vehicle/InitialRot
      mask TypeOptions SampleTime: Simulation 3D Pedestrian/SampleTime | PlantParser/Passenger Vehicle Ray Trace Set/Ts
      mask TypeOptions CoordinateScheme: Simulation 3D Vehicle/CoordinateScheme
      mask Callback VehLightsControl: sim3dblkssharedicon('sim3dblks3dvehterrfbVDBS',gcb,'VehLightsControl');
      mask TypeOptions HeadlightColor: Simulation 3D Vehicle/HeadligtColor
      mask TypeOptions HighBeamIntensity: Simulation 3D Vehicle/HighBeamIntensity
      mask TypeOptions LowBeamIntensity: Simulation 3D Vehicle/LowBeamIntensity
      mask TypeOptions HighBeamConeAngle: Simulation 3D Vehicle/HighBeamRadius
      mask TypeOptions LowBeamConeAngle: Simulation 3D Vehicle/LowBeamRadius
      mask TypeOptions LeftHeadlightOrientation: Simulation 3D Vehicle/LeftHeadlightOrientation
      mask TypeOptions RightHeadlightOrientation: Simulation 3D Vehicle/RightHeadlightOrientation
      mask TypeOptions BrakelightIntensity: Simulation 3D Vehicle/BrakelightIntensity
      mask TypeOptions ReverselightIntensity: Simulation 3D Vehicle/ReverselightIntensity
      mask TypeOptions SignallightIntensity: Simulation 3D Vehicle/IndicatorlightIntensity
      mask TypeOptions SignallightPeriod:
      | Signal Lights Processor/Pulse
      | Generator/Period
      mask TypeOptions SignalPulseWidth:
      | Signal Lights Processor/Pulse
      | Generator/PulseWidth
      mask DialogControl ParameterGroupVar Prompt: shared_sim3dblks:sim3dblkVehicleWithGroundFollowing:blkDlg_ParameterGroupVar
      mask DialogControl PassVehMesh Prompt: Type:
      mask DialogControl PassVehMesh_Internal Prompt: Type:
      mask DialogControl MeshPath Prompt: Path to custom mesh:
      mask DialogControl TrackWidth Prompt: Track width in custom mesh (m):
      mask DialogControl WheelBase Prompt: Wheel base in custom mesh (m):
      mask DialogControl WheelRadius Prompt: Wheel radius in custom mesh (m):
      mask DialogControl VehColor Prompt: Color:
      mask DialogControl VehColor_Internal Prompt: Color:
      mask DialogControl InitialPos Prompt: Initial position [X, Y, Z] (m):
      mask DialogControl InitialRot Prompt: Initial rotation [Roll, Pitch, Yaw] (deg):
      mask DialogControl ActorName Prompt: Name:
      mask DialogControl SampleTime Prompt: Sample time:
      mask DialogControl CoordinateScheme Prompt: CoordinateScheme:
      mask DialogControl VehLightsTab Prompt: shared_sim3dblks:sim3dblkVehicleWithGroundFollowing:blkDg_LightControlsTab
      mask DialogControl VehLightsControl Prompt: Enable light controls:
      mask DialogControl HeadlightSettingsMenu Prompt: shared_sim3dblks:sim3dblkVehicleWithGroundFollowing:blkPrm_HeadlightSettings
      mask DialogControl HeadlightColor Prompt: Headlight color [R,G,B]:
      mask DialogControl HighBeamIntensity Prompt: High beam intensity (cd):
      mask DialogControl LowBeamIntensity Prompt: Low beam intensity (cd):
      mask DialogControl HighBeamConeAngle Prompt: High beam cone half angle (deg):
      mask DialogControl LowBeamConeAngle Prompt: Low beam cone half angle (deg):
      mask DialogControl LeftHeadlightOrientation Prompt: Left headlight beam orientation [Pitch, Yaw] (deg):
      mask DialogControl RightHeadlightOrientation Prompt: Right headlight beam orientation [Pitch, Yaw] (deg):
      mask DialogControl BrakelightSettingsMenu Prompt: shared_sim3dblks:sim3dblkVehicleWithGroundFollowing:blkPrm_BrakelightSettings
      mask DialogControl BrakelightIntensity Prompt: Brake light intensity (cd/m^2):
      mask DialogControl ReverselightSettingsMenu Prompt: shared_sim3dblks:sim3dblkVehicleWithGroundFollowing:blkPrm_ReverselightSettings
      mask DialogControl ReverselightIntensity Prompt: Reverse light intensity (cd/m^2):
      mask DialogControl SignallightSettingsMenu Prompt: shared_sim3dblks:sim3dblkVehicleWithGroundFollowing:blkPrm_SignallightSettings
      mask DialogControl SignallightIntensity Prompt: Turn signal light intensity (cd/m^2):
      mask DialogControl SignallightPeriod Prompt: Period (s):
      mask DialogControl SignalPulseWidth Prompt: Pulse width (% of period):
      mask DialogControl GroundTruthVar Prompt: shared_sim3dblks:sim3dblkVehicleWithGroundFollowing:blkDlg_GroundTruthVar
      mask DialogControl TransformOutportEnabled Prompt: Output location (m) and orientation (rad)
      mask Display:
      | IconInfo = sim3dblkssharedicon('sim3dblks3dvehterrfb', gcb, 'DrawCommands');
      | 
      | image(IconInfo.image, IconInfo.position);
      | 
      | for i = 1:numel(IconInfo.lconn)
      |     port_label('lconn', i, IconInfo.lconn{i})
      | end
      | 
      | for j = 1:numel(IconInfo.rconn)
      |     port_label('rconn', j, IconInfo.rconn{j})
      | end
      | 
      | for k = 1:numel(IconInfo.input)
      |     port_label('input', k, IconInfo.input{k})
      | end
      | 
      | for m = 1:numel(IconInfo.output)
      |     port_label('output', m, IconInfo.output{m})
      | end

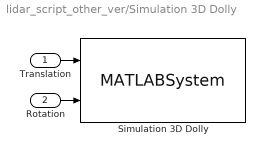
== system lidar_script_other_ver/Simulation 3D Dolly ==
  Translation : Inport
  Rotation : Inport  Port=2
  Simulation 3D Dolly : MATLABSystem  System=Simulation3DDolly  Translation=Translation  Rotation=Rotation  Scale=Scale  Mesh=One-axle dolly  SampleTime=SampleTime
      mask Type: Simulation3DDolly
      mask Display:
      | disp('Dolly');
      | port_label('input',1,'translation');
      | port_label('input',2,'rotation');
  wires:
  Translation/1 -> Simulation 3D Dolly/1
  Rotation/1 -> Simulation 3D Dolly/2

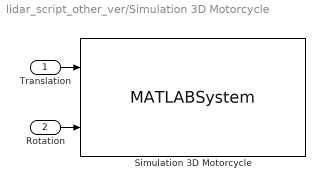
== system lidar_script_other_ver/Simulation 3D Motorcycle ==
  Translation : Inport
  Rotation : Inport  Port=2
  Simulation 3D Motorcycle : MATLABSystem  System=Simulation3DMotorcycle  Translation=Translation  Rotation=Rotation  Scale=ones( 5, 3 )  Mesh=Sports bike  MotorcycleColor=Red  SampleTime=SampleTime
      mask Type: Simulation3DMotorcycle
      mask Display:
      | disp('Motorcycle');
      | port_label('input',1,'translation');
      | port_label('input',2,'rotation');
  wires:
  Rotation/1 -> Simulation 3D Motorcycle/2
  Translation/1 -> Simulation 3D Motorcycle/1

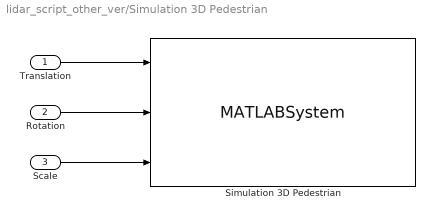
== system lidar_script_other_ver/Simulation 3D Pedestrian ==
  Translation : Inport  Unit=m
  Rotation : Inport  Port=2  Unit=m
  Scale : Inport  Port=3  Unit=deg
  Simulation 3D Pedestrian : MATLABSystem  System=Simulation3DPedestrian  PedestrianType=human_01  SkinTone=Red  HairColor=Red  ZoffsetPos=ZoffsetPos  ActorTag=Pedestrian1  SampleTime=SampleTime
      mask Type: Simulation3DPedestrian
      mask Display:
      | disp('Pedestrian');
      | port_label('input',1,'translation');
      | port_label('input',2,'rotation');
      | port_label('input',3,'scale');
  wires:
  Scale/1 -> Simulation 3D Pedestrian/3
  Rotation/1 -> Simulation 3D Pedestrian/2
  Translation/1 -> Simulation 3D Pedestrian/1

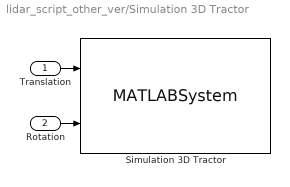
== system lidar_script_other_ver/Simulation 3D Tractor ==
  Translation : Inport
  Rotation : Inport  Port=2
  Simulation 3D Tractor : MATLABSystem  System=Simulation3DTractor  Translation=Translation  Rotation=Rotation  Mesh=Conventional tractor  TractorColor=Red  SampleTime=SampleTime
      mask Type: Simulation3DTractor
      mask Display:
      | disp('Tractor');
      | port_label('input',1,'translation');
      | port_label('input',2,'rotation');
  wires:
  Rotation/1 -> Simulation 3D Tractor/2
  Translation/1 -> Simulation 3D Tractor/1

== system lidar_script_other_ver/Simulation 3D Trailer ==
  Translation : Inport
  Rotation : Inport  Port=2
  Simulation 3D Trailer : MATLABSystem  System=Simulation3DTrailer  Translation=Translation  Rotation=Rotation  Mesh=Two-axle trailer  SampleTime=SampleTime
      mask Type: Simulation3DTrailer
      mask Display:
      | disp('Trailer');
      | port_label('input',1,'translation');
      | port_label('input',2,'rotation');
  wires:
  Rotation/1 -> Simulation 3D Trailer/2
  Translation/1 -> Simulation 3D Trailer/1

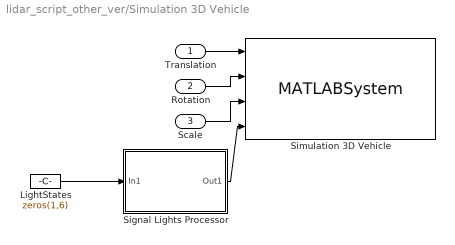
== system lidar_script_other_ver/Simulation 3D Vehicle ==
  Translation : Inport
  Rotation : Inport  Port=2
  Scale : Inport  Port=3
  LightStates : Constant  Value=zeros(1,6)
  Signal Lights Processor : Subsystem
  Simulation 3D Vehicle : MATLABSystem  System=Simulation3DVehicle  Translation=Translation  Rotation=Rotation  Scale=Scale  PassVehMesh=Muscle car  VehColor=Red  MeshPath=/MathWorksSimulation/Vehicles/Muscle/Meshes/SK_MuscleCar.SK_MuscleCar  EnableLightControls=false  LeftHeadlightOrientation=LeftHeadlightOrientation  LeftHeadlightLocation=[ 50, 0, 0 ]  RightHeadlightOrientation=RightHeadlightOrientation  RightHeadlightLocation=[ 50, 0, 0 ]  HeadligtColor=HeadlightColor  TaillightColor=[1 0 0]  BrakelightColor=[ 1, 0, 0 ]  ReverselightColor=[ 1, 0.868, 0.3234 ]  SignallightColor=[ 1, 0.146, 0 ]  HighBeamIntensity=HighBeamIntensity  LowBeamIntensity=LowBeamIntensity  AttenuationRadius=10000  HighBeamRadius=HighBeamConeAngle  LowBeamRadius=LowBeamConeAngle  BrakelightIntensity=BrakelightIntensity  ReverselightIntensity=ReverselightIntensity  IndicatorlightIntensity=SignallightIntensity  MatPath=/MathWorksSimulation/VehicleCommon/Materials/Lights/M_VehicleMatLight.M_VehicleMatLight  SampleTime=SampleTime
      mask Type: Simulation3DVehicle
      mask Display:
      | disp('Vehicle');
      | port_label('input',1,'translation');
      | port_label('input',2,'rotation');
      | port_label('input',3,'scale');
      | port_label('input',4,'LightStates');
  wires:
  Rotation/1 -> Simulation 3D Vehicle/2
  Translation/1 -> Simulation 3D Vehicle/1
  Scale/1 -> Simulation 3D Vehicle/3
  Signal Lights Processor/1(Out1) -> Simulation 3D Vehicle/4
  LightStates/1 -> Signal Lights Processor/1(In1)

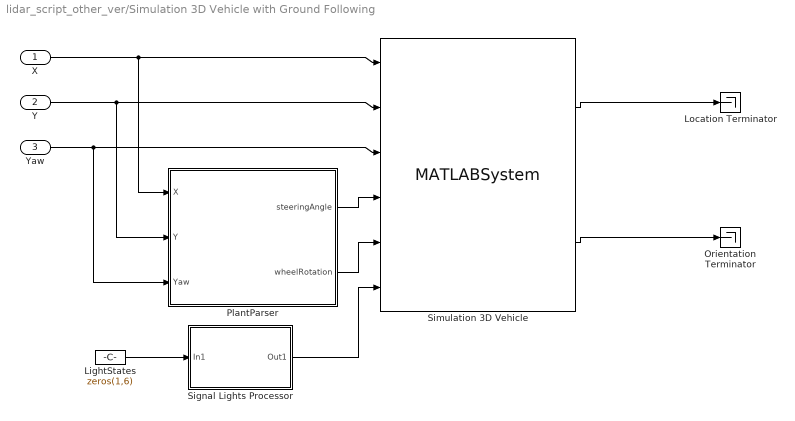
== system lidar_script_other_ver/Simulation 3D Vehicle with Ground Following ==
  X : Inport  Unit=m
  Y : Inport  Port=2  Unit=m
  Yaw : Inport  Port=3  Unit=deg
  LightStates : Constant  Value=zeros(1,6)
  Location Terminator : Terminator
  Orientation Terminator : Terminator
  PlantParser : Subsystem
  Signal Lights Processor : Subsystem
  Simulation 3D Vehicle : MATLABSystem  System=Simulation3DVehicleTerrainFb  PassVehMesh=Muscle car  VehColor=Red  InitialPos=InitialPos  InitialRot=InitialRot  ActorTag=SimulinkVehicle1  CoordinateScheme=ISO  MeshPath=/MathWorksSimulation/Vehicles/Muscle/Meshes/SK_MuscleCar.SK_MuscleCar  TrackWidth=1.9  WheelBase=3  WheelRadius=0.35  EnableLightControls=false  LeftHeadlightOrientation=LeftHeadlightOrientation  LeftHeadlightLocation=[ 50, 0, 0 ]  RightHeadlightOrientation=RightHeadlightOrientation  RightHeadlightLocation=[ 50, 0, 0 ]  HeadligtColor=HeadlightColor  TaillightColor=[1 0 0]  BrakelightColor=[ 1, 0, 0 ]  ReverselightColor=[ 1, 0.868, 0.3234 ]  SignallightColor=[ 1, 0.146, 0 ]  HighBeamIntensity=HighBeamIntensity  LowBeamIntensity=LowBeamIntensity  AttenuationRadius=10000  HighBeamRadius=HighBeamConeAngle  LowBeamRadius=LowBeamConeAngle  BrakelightIntensity=BrakelightIntensity  ReverselightIntensity=ReverselightIntensity  IndicatorlightIntensity=SignallightIntensity  MatPath=/MathWorksSimulation/VehicleCommon/Materials/Lights/M_VehicleMatLight.M_VehicleMatLight  SampleTime=SampleTime
      mask Type: Simulation3DVehicleTerrainFb
      mask Display:
      | disp('Vehicle');
      | port_label('input',1,'X');
      | port_label('input',2,'Y');
      | port_label('input',3,'Yaw');
      | port_label('input',4,'steerAngle');
      | port_label('input',5,'wheelRotation');
      | port_label('input',6,'LightStates');
      | port_label('output',1,'Translation');
      | port_label('output',2,'Rotation');
  wires:
  PlantParser/1(steeringAngle) -> Simulation 3D Vehicle/4
  X/1 -> PlantParser/1(X), Simulation 3D Vehicle/1
  Y/1 -> PlantParser/2(Y), Simulation 3D Vehicle/2
  Yaw/1 -> PlantParser/3(Yaw), Simulation 3D Vehicle/3
  Simulation 3D Vehicle/1 -> Location Terminator/1
  Simulation 3D Vehicle/2 -> Orientation Terminator/1
  PlantParser/2(wheelRotation) -> Simulation 3D Vehicle/5
  Signal Lights Processor/1(Out1) -> Simulation 3D Vehicle/6
  LightStates/1 -> Signal Lights Processor/1(In1)

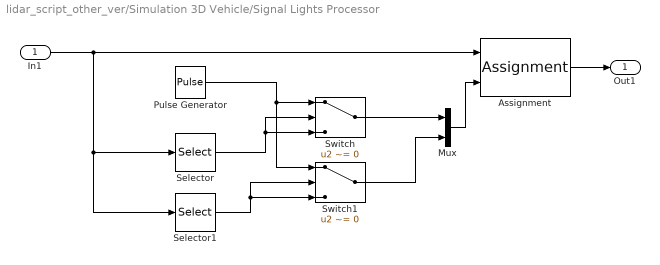
== system lidar_script_other_ver/Simulation 3D Vehicle/Signal Lights Processor ==
  In1 : Inport
  Assignment : Assignment  DiagnosticForDimensions=Warning  IndexOptions=Index vector (dialog)  Indices=[5 6]  OutputSizes=1
  Mux : Mux  Inputs=2
  Pulse Generator : DiscretePulseGenerator  PulseType=Time based  Amplitude=true  Period=SignallightPeriod  PulseWidth=SignalPulseWidth
  Selector : Selector  InputPortWidth=6  IndexOptions=Index vector (dialog)  Indices=[5]  OutputSizes=1
  Selector1 : Selector  InputPortWidth=6  IndexOptions=Index vector (dialog)  Indices=[6]  OutputSizes=1
  Switch : Switch  Criteria=u2 ~= 0
  Switch1 : Switch  Criteria=u2 ~= 0
  Out1 : Outport
  wires:
  Switch1/1 -> Mux/2
  Mux/1 -> Assignment/2
  Assignment/1 -> Out1/1
  In1/1 -> Selector/1, Selector1/1, Assignment/1
  Selector1/1 -> Switch1/2, Switch1/3
  Selector/1 -> Switch/2, Switch/3
  Pulse Generator/1 -> Switch1/1, Switch/1
  Switch/1 -> Mux/1

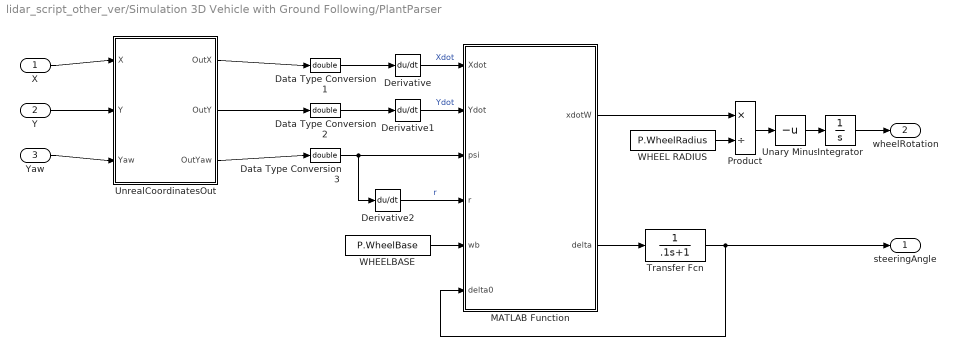
== system lidar_script_other_ver/Simulation 3D Vehicle with Ground Following/PlantParser ==
  X : Inport
  Y : Inport  Port=2
  Yaw : Inport  Port=3
  Data Type Conversion1 : DataTypeConversion  OutDataTypeStr=double
  Data Type Conversion2 : DataTypeConversion  OutDataTypeStr=double
  Data Type Conversion3 : DataTypeConversion  OutDataTypeStr=double
  Derivative : Derivative  CoefficientInTFapproximation=1e-3
  Derivative1 : Derivative  CoefficientInTFapproximation=1e-3
  Derivative2 : Derivative  CoefficientInTFapproximation=1e-3
  Integrator : Integrator  WrapState=on  WrappedStateUpperValue=2*pi  WrappedStateLowerValue=0  ZeroCross=off
  MATLAB Function : MATLAB Function  TreatAsAtomicUnit=on
  Product : Product  Inputs=*/
  Transfer Fcn : TransferFcn  Denominator=[.1 1]
  Unary Minus : UnaryMinus
  UnrealCoordinatesOut : Subsystem  mask{CoordinateScheme=CoordinateScheme}
  WHEEL RADIUS : Constant  Value=P.WheelRadius  OutDataTypeStr=double
  WHEELBASE : Constant  Value=P.WheelBase  OutDataTypeStr=double
  steeringAngle : Outport  VectorParamsAs1DForOutWhenUnconnected=off
  wheelRotation : Outport  Port=2  VectorParamsAs1DForOutWhenUnconnected=off
  wires:
  Data Type Conversion3/1 -> MATLAB Function/3(psi), Derivative2/1
  Data Type Conversion2/1 -> Derivative1/1
  Data Type Conversion1/1 -> Derivative/1
  Unary Minus/1 -> Integrator/1
  WHEEL RADIUS/1 -> Product/2
  Product/1 -> Unary Minus/1
  WHEELBASE/1 -> MATLAB Function/5(wb)
  Transfer Fcn/1 -> MATLAB Function/6(delta0), steeringAngle/1
  Derivative1/1 -> MATLAB Function/2(Ydot)  "Ydot"
  MATLAB Function/2(delta) -> Transfer Fcn/1
  MATLAB Function/1(xdotW) -> Product/1
  Derivative2/1 -> MATLAB Function/4(r)  "r"
  Derivative/1 -> MATLAB Function/1(Xdot)  "Xdot"
  Integrator/1 -> wheelRotation/1
  UnrealCoordinatesOut/2(OutY) -> Data Type Conversion2/1
  UnrealCoordinatesOut/1(OutX) -> Data Type Conversion1/1
  UnrealCoordinatesOut/3(OutYaw) -> Data Type Conversion3/1
  Yaw/1 -> UnrealCoordinatesOut/3(Yaw)
  Y/1 -> UnrealCoordinatesOut/2(Y)
  X/1 -> UnrealCoordinatesOut/1(X)

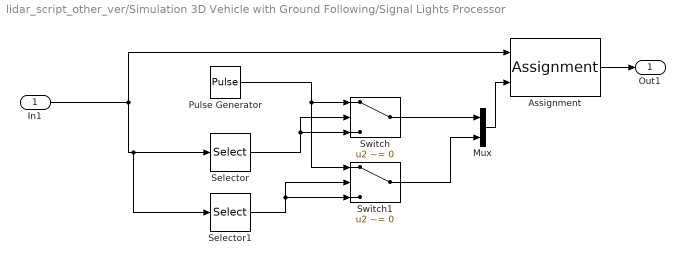
== system lidar_script_other_ver/Simulation 3D Vehicle with Ground Following/Signal Lights Processor ==
  In1 : Inport
  Assignment : Assignment  DiagnosticForDimensions=Warning  IndexOptions=Index vector (dialog)  Indices=[5 6]  OutputSizes=1
  Mux : Mux  Inputs=2
  Pulse Generator : DiscretePulseGenerator  PulseType=Time based  Amplitude=true  Period=SignallightPeriod  PulseWidth=SignalPulseWidth
  Selector : Selector  InputPortWidth=6  IndexOptions=Index vector (dialog)  Indices=[5]  OutputSizes=1
  Selector1 : Selector  InputPortWidth=6  IndexOptions=Index vector (dialog)  Indices=[6]  OutputSizes=1
  Switch : Switch  Criteria=u2 ~= 0
  Switch1 : Switch  Criteria=u2 ~= 0
  Out1 : Outport
  wires:
  Switch1/1 -> Mux/2
  Mux/1 -> Assignment/2
  Assignment/1 -> Out1/1
  In1/1 -> Selector/1, Selector1/1, Assignment/1
  Selector1/1 -> Switch1/2, Switch1/3
  Selector/1 -> Switch/2, Switch/3
  Pulse Generator/1 -> Switch1/1, Switch/1
  Switch/1 -> Mux/1

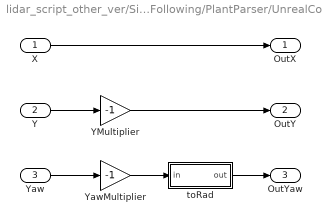
== system lidar_script_other_ver/Simulation 3D Vehicle with Ground Following/PlantParser/UnrealCoordinatesOut ==
  X : Inport
  Y : Inport  Port=2
  Yaw : Inport  Port=3
  YMultiplier : Gain  Gain=-1
  YawMultiplier : Gain  Gain=-1
  toRad : Subsystem
  OutX : Outport  VectorParamsAs1DForOutWhenUnconnected=off
  OutY : Outport  Port=2  VectorParamsAs1DForOutWhenUnconnected=off
  OutYaw : Outport  Port=3  VectorParamsAs1DForOutWhenUnconnected=off
  wires:
  X/1 -> OutX/1
  Y/1 -> YMultiplier/1
  Yaw/1 -> YawMultiplier/1
  YMultiplier/1 -> OutY/1
  YawMultiplier/1 -> toRad/1(in)
  toRad/1(out) -> OutYaw/1

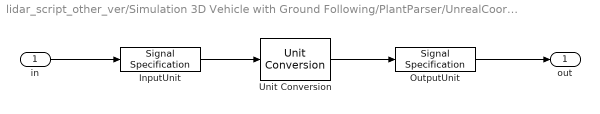
== system lidar_script_other_ver/Simulation 3D Vehicle with Ground Following/PlantParser/UnrealCoordinatesOut/toRad ==
  in : Inport
  InputUnit : SignalSpecification  Unit=deg
  OutputUnit : SignalSpecification  Unit=rad
  Unit Conversion : UnitConversion
  out : Outport  VectorParamsAs1DForOutWhenUnconnected=off
  wires:
  OutputUnit/1 -> out/1
  in/1 -> InputUnit/1
  Unit Conversion/1 -> OutputUnit/1
  InputUnit/1 -> Unit Conversion/1

== matlab function lidar_script_other_ver/Simulation 3D Vehicle with Ground Following/PlantParser/MATLAB Function ==
  data: Xdot input; xdotW output; Ydot input; psi input; r input; wb input; delta0 input; delta output
function [xdotW, delta] = WheelEstimation(Xdot, Ydot, psi, r, wb, delta0)
    [xdotW, delta] = wheelEstCalc(Xdot, Ydot, psi, r, wb, delta0);
end
